simulink model "soft_switch_new_simulation_4"  (R2025b)
settings: Solver=ode15s  StartTime=0.0  StopTime=0.15  MaxStep=1e-5  RelTol=1e-5
InitFcn:
  | % run param_file.m
values from neighbouring files (symbols this model uses):
  opening_ratio = open_ratio_array(k)    [loss_vs_freq_faster.m]
  param = struct()    [Copy_of_param_file.m]    (also in param_file.m; param_file_loss_vs_freq.m; param_file_original.m; param_file_turbine.m)
settings Model: Creator=user  LastModifiedBy=user

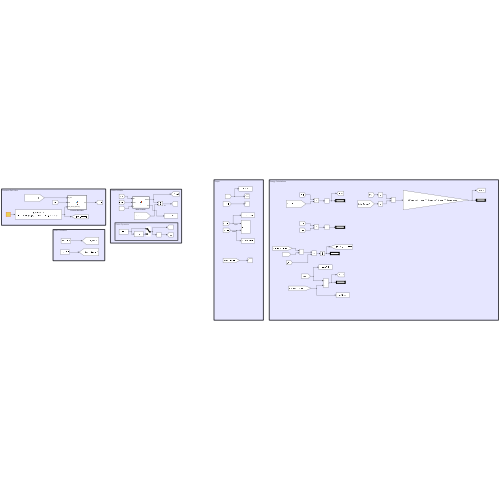
[thumbnail: Simulink's stored preview of the top-level diagram]
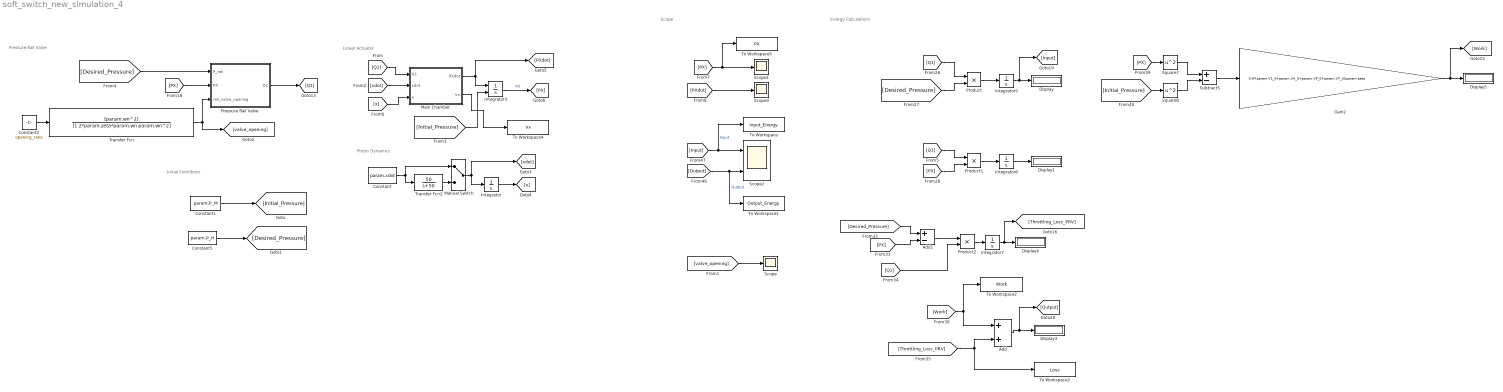
== system soft_switch_new_simulation_4 ==
  note: Piston Dynamics
  note: Energy Calculations
  note: Pressure Rail Valve
  note: Scope
  note: Initial Conditions
  note: Linear Actuator
  Add : Sum
  Add1 : Sum  Inputs=+-
  Constant : Constant  Value=param.xdot
  Constant1 : Constant  Value=param.P_M
  Constant2 : Constant  Value=opening_ratio
  Constant5 : Constant  Value=param.P_H
  Display{,1,3..5} (5 alike) : Display
  Gain2 : Gain  Gain=0.5*(param.V1_0+param.VA_0+param.VP_0+param.VT_0)/param.beta
  Integrator{,5..7} (4 alike) : Integrator
  Integrator3 : Integrator  InitialConditionSource=external
  Main Chamber : MATLAB Function  TreatAsAtomicUnit=on
  Manual Switch : ManualSwitch
  Pressure Rail Valve : MATLAB Function  TreatAsAtomicUnit=on
  Product : Product
  Product1 : Product
  Product2 : Product
  Scope : Scope
      settings: ActiveDisplayYMinimum=-1  ActiveDisplayYMaximum=1
  Scope1 : Scope
      settings: ActiveDisplayYMinimum=2.6711470255232407E+6  ActiveDisplayYMaximum=1.041774547585508E+7  DataLoggingVariableName=ScopeData2
  Scope2 : Scope  NumInputPorts=2
      settings: ActiveDisplayYMinimum=-1.034828401643223  ActiveDisplayYMaximum=9.3134556147890084
  Scope3 : Scope
      settings: ActiveDisplayYMinimum=2.6711470255232407E+6  ActiveDisplayYMaximum=1.041774547585508E+7  DataLoggingVariableName=ScopeData3
  Square7 : Math  Operator=square
  Square8 : Math  Operator=square
  Subtract5 : Sum  Inputs=+-
  To Workspace : ToWorkspace  VariableName=Input_Energy  SaveFormat=Timeseries  SampleTime=-1
  To Workspace1 : ToWorkspace  VariableName=Output_Energy  SaveFormat=Timeseries  SampleTime=-1
  To Workspace2 : ToWorkspace  VariableName=Work  SaveFormat=Timeseries  SampleTime=-1
  To Workspace3 : ToWorkspace  VariableName=Loss  SaveFormat=Timeseries  SampleTime=-1
  To Workspace4 : ToWorkspace  VariableName=Vx  SaveFormat=Timeseries  SampleTime=-1
  To Workspace5 : ToWorkspace  VariableName=PX  SaveFormat=Timeseries  SampleTime=-1
  Transfer Fcn : TransferFcn  Numerator=[param.wn^2]  Denominator=[1 2*param.zeta*param.wn param.wn^2]
  Transfer Fcn2 : TransferFcn  Numerator=50  Denominator=[1 50]
  wires:
  [Desired_Pressure] -> Pressure Rail Valve/1(P_rail)
  Pressure Rail Valve/1(Q1) -> [Q1]
  Constant1/1 -> [Initial_Pressure]
  Main Chamber/1(PXdot) -> [PXdot], Integrator3/1
  [Initial_Pressure] -> Integrator3/2
  Integrator3/1 -> [PX]  "PX"
  Constant5/1 -> [Desired_Pressure]
  [Q1] -> Main Chamber/1(Q1)
  [PX] -> Pressure Rail Valve/2(PX)
  [Q1] -> Product/1
  [Desired_Pressure] -> Product/2
  Product/1 -> Integrator5/1
  [Q1] -> Product1/1
  [PX] -> Product1/2
  Product1/1 -> Integrator6/1
  Integrator5/1 -> [Input], Display/1
  Integrator6/1 -> Display1/1
  [Work] -> To Workspace2/1, Add/1
  Add/1 -> [Output], Display3/1
  [Desired_Pressure] -> Add1/1
  [PX] -> Add1/2
  Add1/1 -> Product2/1
  [Q1] -> Product2/2
  Product2/1 -> Integrator7/1
  Integrator7/1 -> [Throttling_Loss_PRV], Display4/1
  Subtract5/1 -> Gain2/1
  Gain2/1 -> [Work], Display5/1
  [PX] -> Square7/1
  [Initial_Pressure] -> Square8/1
  Square7/1 -> Subtract5/1
  Square8/1 -> Subtract5/2
  [Input] -> To Workspace/1, Scope2/1  "Input"
  [Output] -> To Workspace1/1, Scope2/2  "Output"
  [Throttling_Loss_PRV] -> To Workspace3/1, Add/2
  Constant2/1 -> Transfer Fcn/1
  Transfer Fcn/1 -> Pressure Rail Valve/3(rail_valve_opening), [valve_opening]
  [valve_opening] -> Scope/1
  [xdot] -> Main Chamber/2(xdot)
  Integrator/1 -> [x]
  [x] -> Main Chamber/3(x)
  Main Chamber/2(Vx) -> To Workspace4/1
  [PX] -> To Workspace5/1, Scope1/1
  [PXdot] -> Scope3/1
  Constant/1 -> Transfer Fcn2/1, Manual Switch/1
  Transfer Fcn2/1 -> Manual Switch/2
  Manual Switch/1 -> Integrator/1, [xdot]

== matlab function soft_switch_new_simulation_4/Pressure Rail Valve ==
  data: P_rail input; Q1 output; PX input; param parameter; rail_valve_opening input
function Q1 = fcn(P_rail,PX,param,rail_valve_opening)

Q1 = param.Cd*rail_valve_opening*param.max_Avt*sqrt(2/param.rho)...
    *sqrt(abs(P_rail-PX))*sign(P_rail-PX);

== matlab function soft_switch_new_simulation_4/Main Chamber ==
  data: Q1 input; xdot input; x input; PXdot output; param parameter; Vx output
function [PXdot, Vx] = fcn(Q1, xdot, x, param)

Vx = param.V1_0+param.VA_0+param.VP_0+param.VT_0+param.Acap*x;
PXdot = (param.beta/Vx)*(Q1-param.Acap*xdot);
